simulink model "VTOLfeedback_sim"  (R2016b)
settings: Solver=ode45  StartTime=0.0  StopTime=300  RelTol=1e-3  EnableMultiTasking=on
InitFcn:
  | param
undefined symbols (not defined in the file or in its folder): drawVTOLsys, P, VTOL_ctrl
settings Model: Creator=beard  LastModifiedBy=Jacob
settings DataIOCC: LimitDataPoints=on  SaveFormat=Array  SignalLoggingSaveFormat=ModelDataLogs
settings OptimizationCC: ExpressionDepthLimit=2147483647  InitFltsAndDblsToZero=on  LifeSpan=inf
settings DebuggingCC: UnderspecifiedInitializationDetection=Classic  MergeDetectMultiDrivingBlocksExec=none  SolverPrmCheckMsg=warning  FcnCallInpInsideContextMsg=warning  StateNameClashWarn=warning  SFUnexpectedBacktrackingDiag=warning  SFNoUnconditionalDefaultTransitionDiag=warning  SFExecutionAtInitializationDiag=none
settings HardwareCC: ProdBitPerPointer=32  ProdBitPerSizeT=32  ProdBitPerPtrDiffT=32  ProdLargestAtomicFloat=None  ProdIntDivRoundTo=Undefined  ProdEndianess=Unspecified  ProdWordSize=32  ProdHWDeviceType=32-bit Generic
settings ModelReferenceCC: PropagateSignalLabelsOutOfModel=off
settings GRTTargetCC: TargetLangStandard=C89/C90 (ANSI)  GeneratePreprocessorConditionals=Disable all  CombineOutputUpdateFcns=off  GRTInterface=on
settings ConfigComp: CovMetricSettings=dw  CovHtmlReporting=on  CovSaveCumulativeToWorkspaceVar=on  CovSaveSingleToWorkspaceVar=on  CovExternalEMLEnable=off

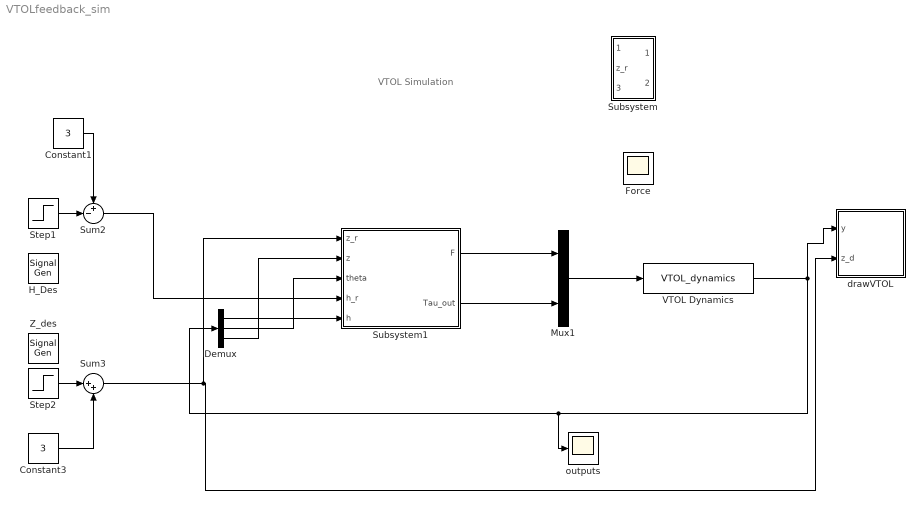
== system VTOLfeedback_sim ==
  note: VTOL Simulation
  Constant1 : Constant  Value=3
  Constant3 : Constant  Value=3
  Demux : Demux  Outputs=3
  Force : Scope
  H_Des : SignalGenerator  WaveForm=square  Amplitude=2  Frequency=.2  Units=rad/sec
  Mux1 : Mux  Inputs=2
  Step1 : Step  After=2  SampleTime=0
  Step2 : Step  After=2  SampleTime=0
  Subsystem : Subsystem
  Subsystem1 : Subsystem
  Sum2 : Sum  Inputs=+-|
  Sum3 : Sum  Inputs=|++
  VTOL Dynamics : S-Function  FunctionName=VTOL_dynamics  Parameters=P  SFunctionDeploymentMode=off  EnableBusSupport=off
  Z_des : SignalGenerator  WaveForm=square  Amplitude=2.5  Frequency=.08  Units=rad/sec
  drawVTOL : Subsystem
      mask Display: image(imread('tv.jpg'))
  "outputs " : Scope
  wires:
  Constant1/1 -> Sum2/1
  Mux1/1 -> VTOL Dynamics/1
  Constant3/1 -> Sum3/2
  VTOL Dynamics/1 -> Demux/1, "outputs "/1, drawVTOL/1(y)
  Sum3/1 -> Subsystem1/1(z_r), drawVTOL/2("z_d ")
  Sum2/1 -> Subsystem1/4(h_r)
  Demux/1 -> Subsystem1/5(h)
  Demux/2 -> Subsystem1/3(theta)
  Demux/3 -> Subsystem1/2(z)
  Subsystem1/1(F) -> Mux1/1
  Subsystem1/2(Tau_out) -> Mux1/2
  Step1/1 -> Sum2/2
  Step2/1 -> Sum3/1

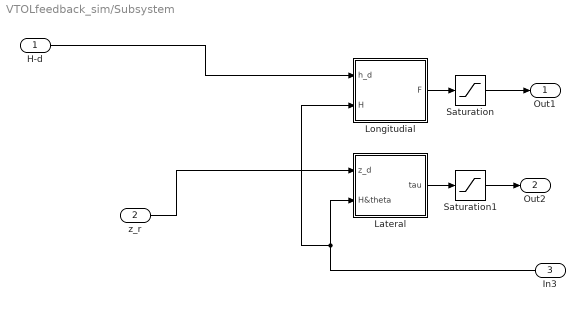
== system VTOLfeedback_sim/Subsystem ==
  "H-d " : Inport
  z_r : Inport  Port=2
  In3 : Inport  Port=3
  Lateral : Subsystem
  Longitudial : Subsystem
  Saturation : Saturate  UpperLimit=30  LowerLimit=0
  Saturation1 : Saturate  UpperLimit=4.5  LowerLimit=-4.5
  Out1 : Outport
  Out2 : Outport  Port=2
  wires:
  Longitudial/1(F) -> Saturation/1
  "H-d "/1 -> Longitudial/1(h_d)
  Saturation1/1 -> Out2/1
  Lateral/1(tau) -> Saturation1/1
  Saturation/1 -> Out1/1
  In3/1 -> Lateral/2(H&theta), Longitudial/2(H)
  z_r/1 -> Lateral/1(z_d)

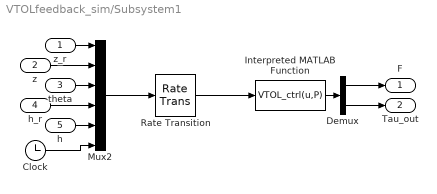
== system VTOLfeedback_sim/Subsystem1 ==
  z_r : Inport
  z : Inport  Port=2
  theta : Inport  Port=3
  h_r : Inport  Port=4
  h : Inport  Port=5
  Clock : Clock
  Demux : Demux  Outputs=2
  Interpreted MATLAB Function : MATLABFcn  MATLABFcn=VTOL_ctrl(u,P)  OutputDimensions=2  Output1D=off
  Mux2 : Mux  Inputs=6
  Rate Transition : RateTransition  OutPortSampleTime=P.Ts
  F : Outport
  Tau_out : Outport  Port=2
  wires:
  Interpreted MATLAB Function/1 -> Demux/1
  h/1 -> Mux2/5
  Demux/1 -> F/1
  theta/1 -> Mux2/3
  h_r/1 -> Mux2/4
  Demux/2 -> Tau_out/1
  Mux2/1 -> Rate Transition/1
  z/1 -> Mux2/2
  z_r/1 -> Mux2/1
  Clock/1 -> Mux2/6
  Rate Transition/1 -> Interpreted MATLAB Function/1

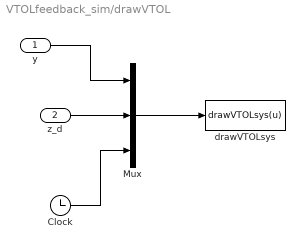
== system VTOLfeedback_sim/drawVTOL ==
  y : Inport
  "z_d " : Inport  Port=2
  Clock : Clock
  Mux : Mux  Inputs=3
  "drawVTOLsys " : MATLABFcn  MATLABFcn=drawVTOLsys(u)  OutputDimensions=0  SampleTime=0.1
  wires:
  Mux/1 -> "drawVTOLsys "/1
  y/1 -> Mux/1
  Clock/1 -> Mux/3
  "z_d "/1 -> Mux/2

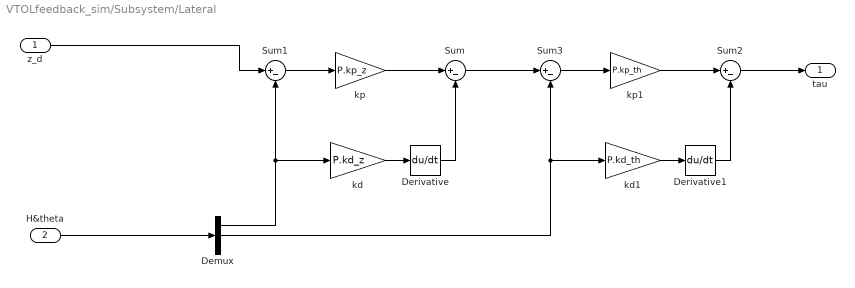
== system VTOLfeedback_sim/Subsystem/Lateral ==
  z_d : Inport
  H&theta : Inport  Port=2
  Demux : Demux  Outputs=3
  Derivative : Derivative
  Derivative1 : Derivative
  Sum{,1..3} (4 alike) : Sum  Inputs=|+-
  kd : Gain  Gain=P.kd_z
  kd1 : Gain  Gain=P.kd_th
  kp : Gain  Gain=P.kp_z
  kp1 : Gain  Gain=P.kp_th
  tau : Outport
  wires:
  z_d/1 -> Sum1/1
  Sum1/1 -> kp/1
  kd/1 -> Derivative/1
  kp/1 -> Sum/1
  Derivative/1 -> Sum/2
  Sum3/1 -> kp1/1
  kd1/1 -> Derivative1/1
  kp1/1 -> Sum2/1
  Derivative1/1 -> Sum2/2
  Sum/1 -> Sum3/1
  Sum2/1 -> tau/1
  H&theta/1 -> Demux/1
  Demux/2 -> kd1/1, Sum3/2
  Demux/1 -> kd/1, Sum1/2

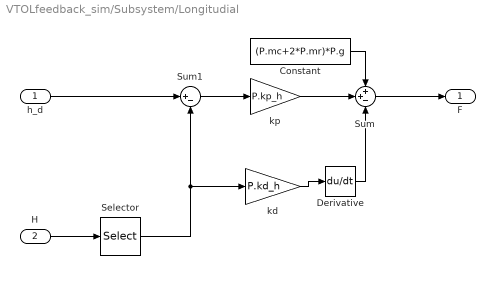
== system VTOLfeedback_sim/Subsystem/Longitudial ==
  h_d : Inport
  H : Inport  Port=2
  Constant : Constant  Value=(P.mc+2*P.mr)*P.g
  Derivative : Derivative
  Selector : Selector  InputPortWidth=3  IndexOptions=Index vector (dialog)  Indices=[3]  OutputSizes=1
  Sum : Sum  Inputs=++-
  Sum1 : Sum  Inputs=|+-
  kd : Gain  Gain=P.kd_h
  kp : Gain  Gain=P.kp_h
  F : Outport
  wires:
  Sum/1 -> F/1
  kp/1 -> Sum/2
  h_d/1 -> Sum1/1
  Sum1/1 -> kp/1
  H/1 -> Selector/1
  Derivative/1 -> Sum/3
  kd/1 -> Derivative/1
  Constant/1 -> Sum/1
  Selector/1 -> Sum1/2, kd/1
